simulink model "FilterRealization"  (R2020b)
settings: Solver=VariableStepAuto  StartTime=0.0  StopTime=50  FixedStep=0.001  RelTol=1e-3
settings Model: Creator=baner  LastModifiedBy=baner

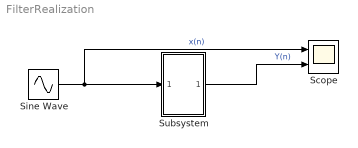
== system FilterRealization ==
  Scope : Scope  NumInputPorts=2
  Sine Wave : Sin  Frequency=10  SampleTime=0
  Subsystem : Subsystem  TreatAsAtomicUnit=on
  wires:
  Sine Wave/1 -> Scope/1, Subsystem/1(x(n))  "x(n)"
  Subsystem/1(y(n)) -> Scope/2  "Y(n)"

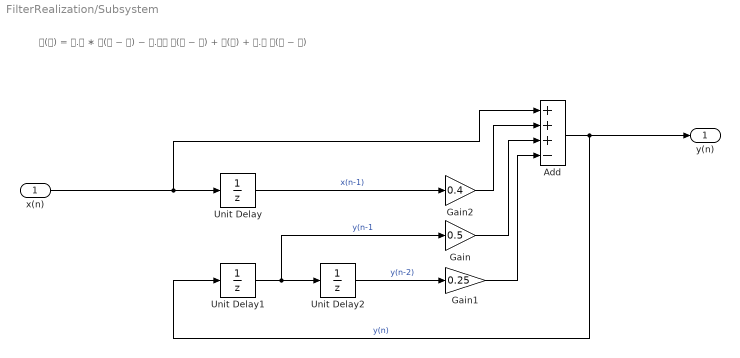
== system FilterRealization/Subsystem ==
  note: 𝐲(𝐧) = 𝟎.𝟓 ∗ 𝐲(𝐧 − 𝟏) − 𝟎.𝟐𝟓 𝐲(𝐧 − 𝟐) + 𝐱(𝐧) + 𝟎.𝟒 𝐱(𝐧 − 𝟏)
  x(n) : Inport
  Add : Sum  Inputs=+++-
  Gain : Gain  Gain=0.5
  Gain1 : Gain  Gain=0.25
  Gain2 : Gain  Gain=0.4
  Unit Delay : UnitDelay  SampleTime=-1  HasFrameUpgradeWarning=on
  Unit Delay1 : UnitDelay  SampleTime=-1  HasFrameUpgradeWarning=on
  Unit Delay2 : UnitDelay  SampleTime=-1  HasFrameUpgradeWarning=on
  y(n) : Outport
  wires:
  Unit Delay/1 -> Gain2/1  "x(n-1)"
  Gain2/1 -> Add/2
  Gain/1 -> Add/3
  Gain1/1 -> Add/4
  Unit Delay2/1 -> Gain1/1  "y(n-2)"
  Unit Delay1/1 -> Gain/1, Unit Delay2/1  "y(n-1"
  Add/1 -> y(n)/1, Unit Delay1/1  "y(n)"
  x(n)/1 -> Add/1, Unit Delay/1
